simulink model "control_system_simulation"  (R2017b)
settings: Solver=VariableStepAuto  StartTime=0.0  StopTime=10.0  RelTol=1e-3
libraries: simulink x4
settings Model: Creator=Alex  LastModifiedBy=Alex

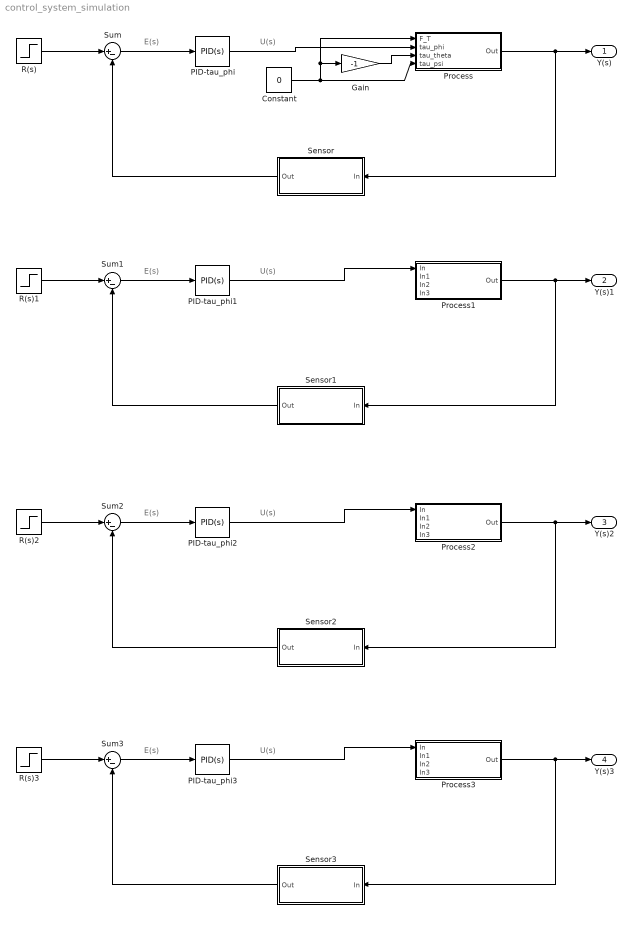
== system control_system_simulation ==
  note: U(s)
  note: E(s)
  note: E(s)
  note: U(s)
  note: E(s)
  note: U(s)
  note: E(s)
  note: U(s)
  Constant : Constant  Value=0
  Gain : Gain  Gain=-1
  PID-tau_phi{,1..3} (4 alike) : simulink/Continuous/PID Controller  Controller=PID  TimeDomain=Continuous-time  SampleTime=-1  IntegratorMethod=Forward Euler  FilterMethod=Forward Euler  Form=Parallel  UseFilter=on  ControllerParametersSource=internal  P=1  I=1  D=0  N=100  InitialConditionSource=internal  InitialConditionForIntegrator=0  InitialConditionForFilter=0  ExternalReset=none  LimitOutput=off  UpperSaturationLimit=inf  LowerSaturationLimit=-inf  LinearizeAsGain=on  AntiWindupMode=none  Kb=1  TrackingMode=off  Kt=1  PParamMin=[]  PParamMax=[]  IParamMin=[]  IParamMax=[]  DParamMin=[]  DParamMax=[]  NParamMin=[]  NParamMax=[]  KbParamMin=[]  KbParamMax=[]  KtParamMin=[]  KtParamMax=[]  POutMin=[]  POutMax=[]  IOutMin=[]  IOutMax=[]  DOutMin=[]  DOutMax=[]  NOutMin=[]  NOutMax=[]  KbOutMin=[]  KbOutMax=[]  KtOutMin=[]  KtOutMax=[]  IntegratorOutMin=[]  IntegratorOutMax=[]  FilterOutMin=[]  FilterOutMax=[]  SumOutMin=[]  SumOutMax=[]  SumI1OutMin=[]  SumI1OutMax=[]  SumI2OutMin=[]  SumI2OutMax=[]  SumI3OutMin=[]  SumI3OutMax=[]  SumDOutMin=[]  SumDOutMax=[]  SaturationOutMin=[]  SaturationOutMax=[]  IntegratorContinuousStateAttributes=''  IntegratorStateMustResolveToSignalObject=off  IntegratorRTWStateStorageClass=Auto  FilterContinuousStateAttributes=''  FilterStateMustResolveToSignalObject=off  FilterRTWStateStorageClass=Auto  DifferentiatorICPrevScaledInput=0  DifferentiatorOutMin=[]  DifferentiatorOutMax=[]  InitialConditionSetting=State (most efficient)  FilterDiffOutCoefMin=[]  FilterDiffOutCoefMax=[]  SumDenOutMin=[]  SumDenOutMax=[]  SumNumOutMin=[]  SumNumOutMax=[]  ReciprocalOutMin=[]  ReciprocalOutMax=[]  DivideOutMin=[]  DivideOutMax=[]  TunerSelectOption=Transfer Function Based (PID Tuner App)
  Process : Subsystem
  Process1 : Subsystem
  Process2 : Subsystem
  Process3 : Subsystem
  R(s){,1..3} (4 alike) : Step  SampleTime=0
  Sensor : Subsystem
  Sensor1 : Subsystem
  Sensor2 : Subsystem
  Sensor3 : Subsystem
  Sum{,1..3} (4 alike) : Sum  Inputs=|+-
  Y(s) : Outport
  Y(s)1 : Outport  Port=2
  Y(s)2 : Outport  Port=3
  Y(s)3 : Outport  Port=4
  wires:
  Sum/1 -> PID-tau_phi/1
  R(s)/1 -> Sum/1
  Process/1(Out) -> Sensor/1(In), Y(s)/1
  Sensor/1(Out) -> Sum/2
  Sensor1/1(Out) -> Sum1/2
  Process1/1(Out) -> Sensor1/1(In), Y(s)1/1
  Sum1/1 -> PID-tau_phi1/1
  PID-tau_phi1/1 -> Process1/1(In)
  R(s)1/1 -> Sum1/1
  Sensor2/1(Out) -> Sum2/2
  Process2/1(Out) -> Sensor2/1(In), Y(s)2/1
  Sum2/1 -> PID-tau_phi2/1
  PID-tau_phi2/1 -> Process2/1(In)
  R(s)2/1 -> Sum2/1
  Sensor3/1(Out) -> Sum3/2
  Process3/1(Out) -> Sensor3/1(In), Y(s)3/1
  Sum3/1 -> PID-tau_phi3/1
  PID-tau_phi3/1 -> Process3/1(In)
  R(s)3/1 -> Sum3/1
  Constant/1 -> Process/1(F_T), Gain/1, Process/4(tau_psi)
  Gain/1 -> Process/3(tau_theta)
  PID-tau_phi/1 -> Process/2(tau_phi)

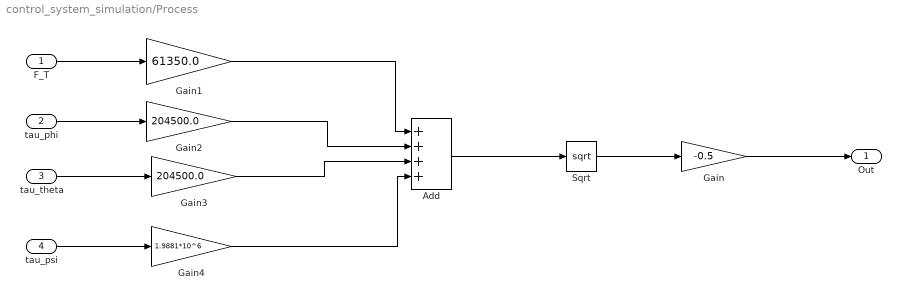
== system control_system_simulation/Process ==
  F_T : Inport
  tau_phi : Inport  Port=2
  tau_theta : Inport  Port=3
  tau_psi : Inport  Port=4
  Add : Sum  Inputs=++++
  Gain : Gain  Gain=-0.5
  Gain1 : Gain  Gain=61350.0
  Gain2 : Gain  Gain=204500.0
  Gain3 : Gain  Gain=204500.0
  Gain4 : Gain  Gain=1.9881*10^6
  Sqrt : Sqrt  SaturateOnIntegerOverflow=on
  Out : Outport
  wires:
  Add/1 -> Sqrt/1
  F_T/1 -> Gain1/1
  tau_phi/1 -> Gain2/1
  tau_theta/1 -> Gain3/1
  tau_psi/1 -> Gain4/1
  Gain1/1 -> Add/1
  Gain2/1 -> Add/2
  Gain3/1 -> Add/3
  Gain4/1 -> Add/4
  Sqrt/1 -> Gain/1
  Gain/1 -> Out/1

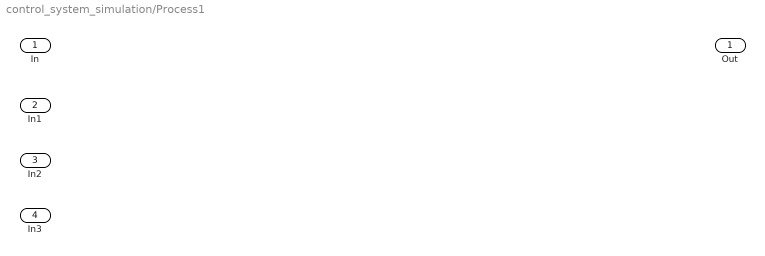
== system control_system_simulation/Process1 ==
  In : Inport
  In1 : Inport  Port=2
  In2 : Inport  Port=3
  In3 : Inport  Port=4
  Out : Outport

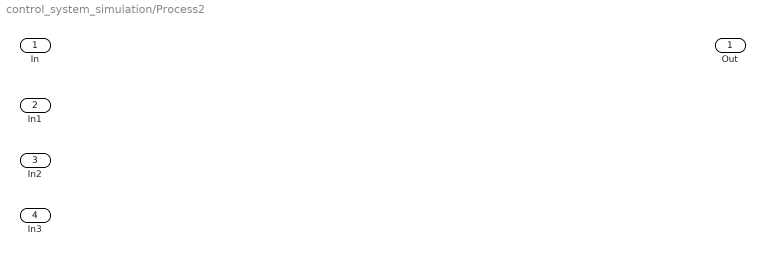
== system control_system_simulation/Process2 ==
  In : Inport
  In1 : Inport  Port=2
  In2 : Inport  Port=3
  In3 : Inport  Port=4
  Out : Outport

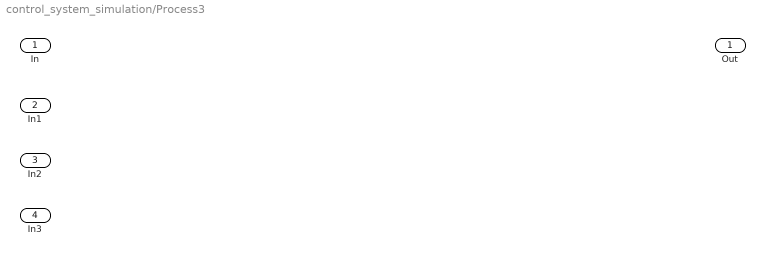
== system control_system_simulation/Process3 ==
  In : Inport
  In1 : Inport  Port=2
  In2 : Inport  Port=3
  In3 : Inport  Port=4
  Out : Outport

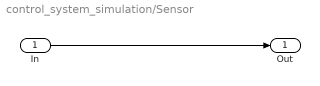
== system control_system_simulation/Sensor ==
  In : Inport
  Out : Outport
  wires:
  In/1 -> Out/1

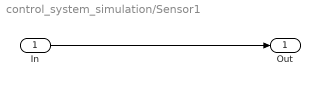
== system control_system_simulation/Sensor1 ==
  In : Inport
  Out : Outport
  wires:
  In/1 -> Out/1

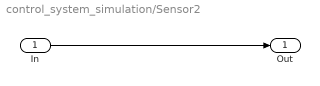
== system control_system_simulation/Sensor2 ==
  In : Inport
  Out : Outport
  wires:
  In/1 -> Out/1

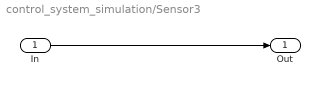
== system control_system_simulation/Sensor3 ==
  In : Inport
  Out : Outport
  wires:
  In/1 -> Out/1
